simulink model "deadtime"  (R2015a)
settings: Solver=ode45  StartTime=0.0  StopTime=10.0  RelTol=1e-3
undefined symbols (not defined in the file): Kimiz5, Kpmiz5
settings Model: Creator=PC  LastModifiedBy=PC

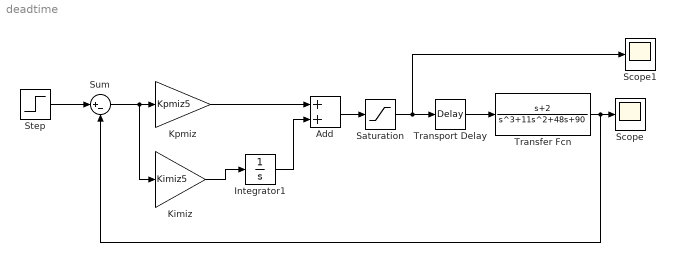
== system deadtime ==
  Add : Sum
  Integrator1 : Integrator
  Kimiz : Gain  Gain=Kimiz5
  Kpmiz : Gain  Gain=Kpmiz5
  Saturation : Saturate  UpperLimit=90  LowerLimit=0
  Scope : Scope
  Scope1 : Scope
  Step : Step  SampleTime=0
  Sum : Sum  Inputs=|+-
  Transfer Fcn : TransferFcn  Numerator=[1 2]  Denominator=[1 11 48 90]
  Transport Delay : TransportDelay  DelayTime=0.01
  wires:
  Sum/1 -> Kpmiz/1, Kimiz/1
  Step/1 -> Sum/1
  Kimiz/1 -> Integrator1/1
  Integrator1/1 -> Add/2
  Kpmiz/1 -> Add/1
  Transfer Fcn/1 -> Sum/2, Scope/1
  Add/1 -> Saturation/1
  Transport Delay/1 -> Transfer Fcn/1
  Saturation/1 -> Transport Delay/1, Scope1/1
